simulink model "motor_model"  (R2022a)
settings: Solver=FixedStepAuto  StartTime=0.0  StopTime=sim_time  FixedStep=0.001  RelTol=1e-3
undefined symbols (not defined in the file or in its folder): den_c, den_sys, num_c, num_sys
libraries: simulink x1, slpidlib x1
settings Model: Creator=michi  LastModifiedBy=michi

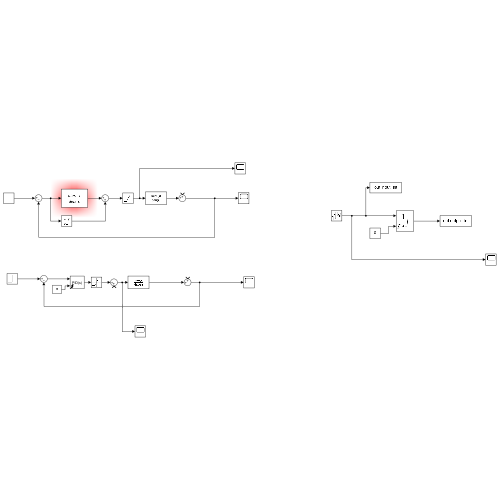
[thumbnail: Simulink's stored preview of the top-level diagram]
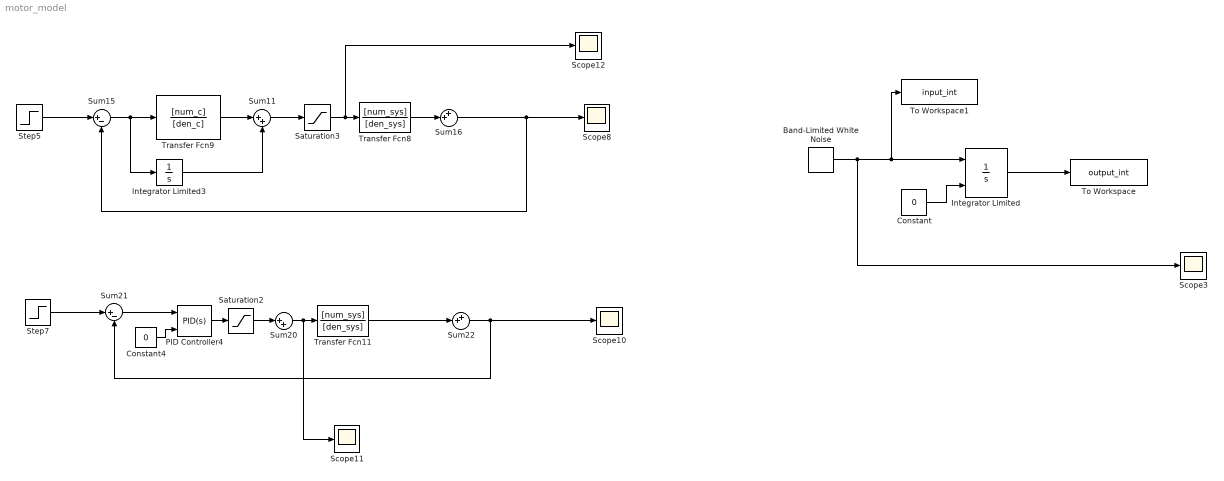
== system motor_model ==
  Band-Limited White Noise : simulink/Sources/Band-Limited White Noise  Cov=[1]  Ts=0.001  seed=[23341]
  Constant : Constant  Value=0
  Constant4 : Constant  Value=0
  Integrator Limited : Integrator  ExternalReset=rising  LimitOutput=on  UpperSaturationLimit=3  LowerSaturationLimit=-3
  Integrator Limited3 : Integrator  LimitOutput=on  UpperSaturationLimit=1  LowerSaturationLimit=0
  PID Controller4 : slpidlib/PID Controller  Controller=PID  Form=Ideal  TimeDomain=Continuous-time  UseExternalTs=off  SampleTime=-1  IntegratorMethod=Forward Euler  FilterMethod=Forward Euler  ControllerParametersSource=internal  P=10  I=0.04  UseKiTs=off  D=10  N=100  UseFilter=on  TunerSelectOption=Transfer Function Based (PID Tuner App)  InitialConditionSource=internal  InitialConditionForIntegrator=0  InitialConditionForFilter=0  DifferentiatorICPrevScaledInput=0  ExternalReset=rising  TrackingMode=off  Kt=1  LimitOutput=off  SatLimitsSource=internal  UpperSaturationLimit=inf  LowerSaturationLimit=-inf  LinearizeAsGain=on  AntiWindupMode=none  Kb=1  POutMin=[]  POutMax=[]  IOutMin=[]  IOutMax=[]  DOutMin=[]  DOutMax=[]  NOutMin=[]  NOutMax=[]  SumOutMin=[]  SumOutMax=[]  SaturationOutMin=[]  SaturationOutMax=[]  PParamMin=[]  PParamMax=[]  IParamMin=[]  IParamMax=[]  DParamMin=[]  DParamMax=[]  NParamMin=[]  NParamMax=[]  KbParamMin=[]  KbParamMax=[]  KtParamMin=[]  KtParamMax=[]  KbOutMin=[]  KbOutMax=[]  KtOutMin=[]  KtOutMax=[]  IntegratorOutMin=[]  IntegratorOutMax=[]  FilterOutMin=[]  FilterOutMax=[]  SumI1OutMin=[]  SumI1OutMax=[]  SumI2OutMin=[]  SumI2OutMax=[]  SumI3OutMin=[]  SumI3OutMax=[]  SumI4OutMin=[]  SumI4OutMax=[]  SumDOutMin=[]  SumDOutMax=[]  DifferentiatorOutMin=[]  DifferentiatorOutMax=[]  FilterDiffOutCoefMin=[]  FilterDiffOutCoefMax=[]  ReciprocalOutMin=[]  ReciprocalOutMax=[]  SumDenOutMin=[]  SumDenOutMax=[]  SumNumOutMin=[]  SumNumOutMax=[]  DivideOutMin=[]  DivideOutMax=[]  UdiffTsProdOutMin=[]  UdiffTsProdOutMax=[]  NTsProdOutMin=[]  NTsProdOutMax=[]  UintegralTsProdOutMin=[]  UintegralTsProdOutMax=[]  UngainTsProdOutMin=[]  UngainTsProdOutMax=[]  IntegratorContinuousStateAttributes=''  IntegratorStateMustResolveToSignalObject=off  IntegratorRTWStateStorageClass=Auto  FilterContinuousStateAttributes=''  FilterStateMustResolveToSignalObject=off  FilterRTWStateStorageClass=Auto  ParallelPVariant=Passthrough  IdealPVariant=InternalParameters  IVariant=InternalParameters  DVariant=InternalParameters  IntegratorVariant=Continuous  SatVariant=Disabled  AWVariant=Passthrough  PCopyVariant=Disabled  TRVariant=Disabled  FdbkBlocksVariant=Forward  IdealPFdbkVariant=Disabled  SatFdbkVariant=Disabled  DerivativeFilterVariant=ContFilter  NVariant=InternalParameters  NCopyVariant=Disabled  FilterICVariant=InternalICsFilter  IntegratorICVariant=InternalICs  ExternalResetVariant=ExternalReset  TRSumVariant=Passthrough  SumFdbkVariant=Disabled  SumVariant=Sum_PID  TsampFilterVariant=InternalTs  TsampNgainVariant=Passthrough  TsampIntegralVariant=Passthrough  ExternalSaturationOutDataTypeStr=Inherit: Same as second input  aMode=0
  Saturation2 : Saturate  UpperLimit=3  LowerLimit=-3
  Saturation3 : Saturate  UpperLimit=3  LowerLimit=-3
  Scope{3,8,10..12} (5 alike) : Scope
  Step5 : Step  Time=2  SampleTime=0
  Step7 : Step  Time=2  SampleTime=0
  Sum11 : Sum  Inputs=|++
  Sum15 : Sum  Inputs=|+-
  Sum16 : Sum  Inputs=++|
  Sum20 : Sum  Inputs=|++
  Sum21 : Sum  Inputs=|+-
  Sum22 : Sum  Inputs=++|
  To Workspace : ToWorkspace  VariableName=output_int  SampleTime=-1
  To Workspace1 : ToWorkspace  VariableName=input_int  SampleTime=-1
  Transfer Fcn11 : TransferFcn  Numerator=[num_sys]  Denominator=[den_sys]
  Transfer Fcn8 : TransferFcn  Numerator=[num_sys]  Denominator=[den_sys]
  Transfer Fcn9 : TransferFcn  Numerator=[num_c]  Denominator=[den_c]
  wires:
  Constant/1 -> Integrator Limited/2
  Band-Limited White Noise/1 -> Scope3/1, To Workspace1/1, Integrator Limited/1
  Integrator Limited/1 -> To Workspace/1
  Transfer Fcn9/1 -> Sum11/1
  Sum15/1 -> Transfer Fcn9/1, Integrator Limited3/1
  Step5/1 -> Sum15/1
  Sum11/1 -> Saturation3/1
  Transfer Fcn8/1 -> Sum16/2
  Sum16/1 -> Scope8/1, Sum15/2
  PID Controller4/1 -> Saturation2/1
  Sum21/1 -> PID Controller4/1
  Transfer Fcn11/1 -> Sum22/2
  Sum20/1 -> Scope11/1, Transfer Fcn11/1
  Constant4/1 -> PID Controller4/2
  Step7/1 -> Sum21/1
  Saturation2/1 -> Sum20/1
  Sum22/1 -> Scope10/1, Sum21/2
  Saturation3/1 -> Scope12/1, Transfer Fcn8/1
  Integrator Limited3/1 -> Sum11/2
